simulink model "actuator_level_gripper"  (R2013b)
settings: Solver=FixedStepDiscrete  SolverMode=SingleTasking  StartTime=0.0  StopTime=inf  RelTol=1e-3
settings Model: SimulationMode=external  ExtModeTrigDuration=2  Creator=Joshua  LastModifiedBy=Joshua
settings OptimizationCC: OptimizeModelRefInitCode=on  LifeSpan=1
settings DebuggingCC: SolverPrmCheckMsg=none
settings HardwareCC: ProdBitPerInt=16  ProdBitPerPointer=8  ProdIntDivRoundTo=Zero  ProdEndianess=LittleEndian  ProdWordSize=8  ProdHWDeviceType=Atmel->AVR
settings RTWCC: SystemTargetFile=realtime.tlc  GenerateMakefile=off  TemplateMakefile=realtime.tmf  Description=Run on Target Hardware  RTWVerbose=off  ProcessScript=realtime_make_rtw_hook
settings STFCustomTargetCC: TargetLibSuffix=.a  GenerateSampleERTMain=on  ERTCustomFileBanners=on  SupportNonInlinedSFcns=off  SupportVariableSizeSignals=on  MATLABClassNameForMDSCustomization=Simulink.SoftwareTarget.ERTCustomization  GRTInterface=off  SystemTargetFile=realtime.tlc
settings ERTTargetCC: CodeReplacementLibrary=ANSI_C  GenerateSampleERTMain=on  ParMdlRefBuildCompliant=off  CompOptLevelCompliant=off  ConcurrentExecutionCompliant=off  CombineOutputUpdateFcns=off  ERTFirstTimeCompliant=off  SupportContinuousTime=on  SupportVariableSizeSignals=on  ModelStepFunctionPrototypeControlCompliant=off  CPPClassGenCompliant=off  ExtMode=on  ExtModeTransport=3  ExtModeMexArgs=0 28 115200 30  InlinedParameterPlacement=NonHierarchical  ERTSrcFileBannerTemplate=realtime_code_template.cgt  ERTHdrFileBannerTemplate=realtime_code_template.cgt  ERTDataSrcFileTemplate=realtime_code_template.cgt  ERTDataHdrFileTemplate=realtime_code_template.cgt  ERTCustomFileTemplate=realtime_file_process.tlc

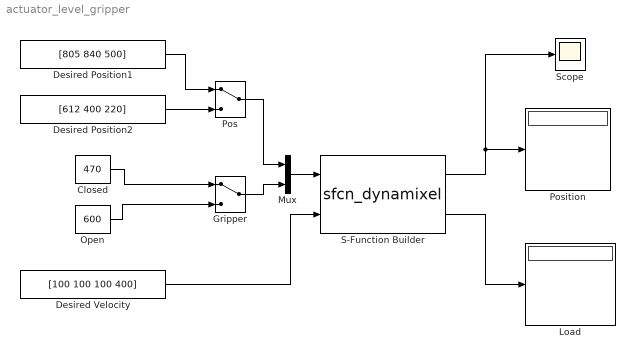
== system actuator_level_gripper ==
  Closed : Constant  Value=470  OutDataTypeStr=int16
  Desired Position1 : Constant  Value=[805 840 500]  OutDataTypeStr=int16
  Desired Position2 : Constant  Value=[612 400 220]  OutDataTypeStr=int16
  Desired Velocity : Constant  Value=[100 100 100 400]  OutDataTypeStr=int16
  Gripper : ManualSwitch
  Load : Display
  Mux : Mux  Inputs=2
  Open : Constant  Value=600  OutDataTypeStr=int16
  Pos : ManualSwitch
  Position : Display
  S-Function Builder : S-Function  InitFcn=try, set_param(gcb,'FunctionName','sfcn_dynamixel'), end  FunctionName=sfcn_dynamixel  Parameters=int8(2),uint32(1000000),int8([1 2 3 4]),uint32(200)  SFunctionModules=sfcn_dynamixel_wrapper  EnableBusSupport=off  mask(Dynamixel driver){portNumber=Serial Port 2, baudrate=1000000, tx=200, identity=[1 2 3 4]}
      mask prompts: portNumber "Serial Port Number (Arduino Mega 2560):"; baudrate "Baud Rate:"; tx "TX Delay Time:"; identity "ID*:"
      mask help:
      | This block provides a driver to control robots built by Dynamixel servos, with a discrete sample time of 0.05 seconds.
      | The first input "q" represents the desired position.
      | The output shows a column vector with the joint angle of each servo in real time.
      mask init:
      | val = [[.9  0.75 0.75 1 1 .9 .9 1]',[1 1 0.75 0.75 .9 .9 1 .9]'];try , sys = get_param(gcb,'SfunBuilderFcnName');if isempty(sys), sys = get_param(gcb,'FunctionName'); end,catch, sys = get_param(gcb,'FunctionName'); end
      settings: CopyFcn=set_param(gcbh,'LinkStatus','none')  PreSaveFcn=try, set_param(gcb,'FunctionName','sfcn_dynamixel'), end  OpenFcn=sfunctionwizard(gcbh)
      mask TypeOptions portNumber: Serial Port 1 | Serial Port 2 | Serial Port 3
      mask Display: plot(val(:,1),val(:,2)),disp(sys), port_label('input',1,'qd'), port_label('input',2,'dqd'), port_label('output',1,'q'), port_label('output',2,'load')
  Scope : Scope
      settings: YMin=200  YMax=850
  wires:
  S-Function Builder/1 -> Scope/1, Position/1
  Desired Velocity/1 -> S-Function Builder/2
  S-Function Builder/2 -> Load/1
  Desired Position1/1 -> Pos/1
  Desired Position2/1 -> Pos/2
  Closed/1 -> Gripper/1
  Open/1 -> Gripper/2
  Mux/1 -> S-Function Builder/1
  Pos/1 -> Mux/1
  Gripper/1 -> Mux/2
